simulink model "ExampleSubsystem"  (R2015b)
settings: Solver=VariableStepAuto  StartTime=0.0  StopTime=10.0  RelTol=1e-3
libraries: ExampleLibrary x1
settings Model: Creator=u265735  LastModifiedBy=u265735
settings ConfigComp: CovModelRefEnable=Off

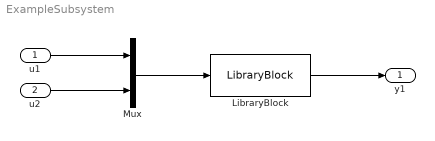
== system ExampleSubsystem ==
  u1 : Inport
  u2 : Inport  Port=2
  LibraryBlock : ExampleLibrary/LibraryBlock
  Mux : Mux  Inputs=2
  y1 : Outport
  wires:
  Mux/1 -> LibraryBlock/1
  u1/1 -> Mux/1
  u2/1 -> Mux/2
  LibraryBlock/1 -> y1/1
